simulink model "RequirementsTable"  (R2022b)
settings: Solver=FixedStepAuto  StartTime=0.0  StopTime=10.0  FixedStep=1e-3  RelTol=1e-3  EnableMultiTasking=on
settings Model: DVExtractedSubsystem=Requirements Table  Creator=coler  LastModifiedBy=coler
settings SolverCC: AlgebraicLoopSolver=TrustRegion
settings OptimizationCC: EnhancedBackFolding=on  PassReuseOutputArgsAs=Individual arguments  ZeroExternalMemoryAtStartup=off  ZeroInternalMemoryAtStartup=off  MaxStackSize=64  OptimizeBlockOrder=speed  DifferentSizesBufferReuse=on  OptimizationCustomize=off  EfficientTunableParamExpr=on
settings DebuggingCC: ParameterTunabilityLossMsg=error  UnconnectedInputMsg=warning  UnconnectedOutputMsg=warning  UnconnectedLineMsg=warning  FrameProcessingCompatibilityMsg=none  SFMachineParentedDataDiag=warning
settings HardwareCC: ProdBitPerPointer=32  ProdBitPerSizeT=32  ProdBitPerPtrDiffT=32  ProdLargestAtomicInteger=Long  ProdLargestAtomicFloat=Double  ProdWordSize=32  ProdHWDeviceType=ARM Compatible->ARM Cortex
settings ModelReferenceCC: EnableRefExpFcnMdlSchedulingChecks=on
settings SFSimCC: MATLABDynamicMemAlloc=off
settings RTWCC: Description=Embedded Coder  SystemTargetFile=ert.tlc  HardwareBoard=NXP FRDM-K64F  TemplateMakefile=ert_default_tmf  Toolchain=GNU Tools for ARM Embedded Processors
settings CodeAppCC: ForceParamTrailComments=on  IgnoreCustomStorageClasses=off  OperatorAnnotations=on  SimulinkDataObjDesc=on  SFDataObjDesc=on  InsertBlockDesc=on
settings ERTTargetCC: ExtMode=on  ExtModeTransport=4  ExtModeMexFile=sendToCommService  ExtModeMexArgs='RA_Modes' 0

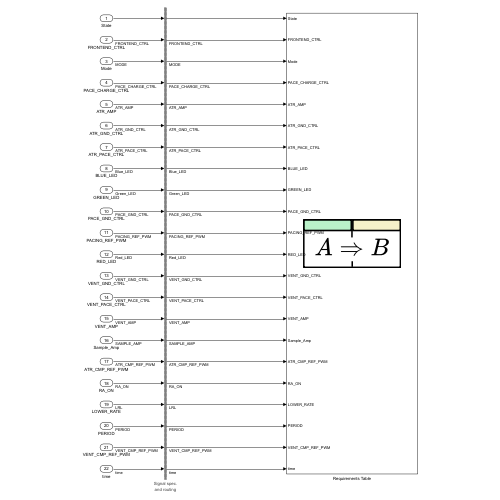
[thumbnail: Simulink's stored preview of the top-level diagram]
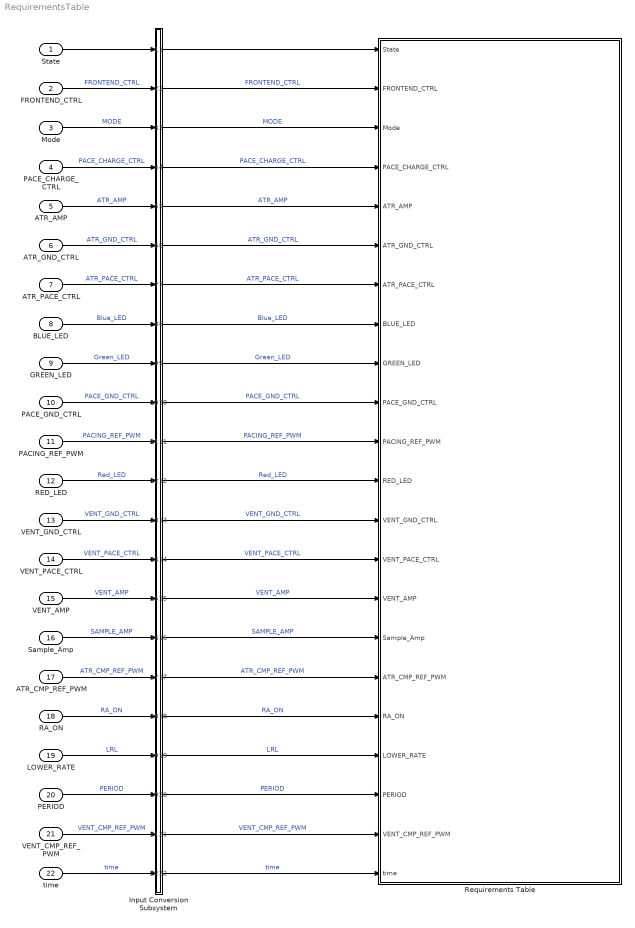
== system RequirementsTable ==
  State : Inport  OutDataTypeStr=double  PortDimensions=[1]  SampleTime=[-1, 0]  Interpolate=off
  FRONTEND_CTRL : Inport  Port=2  OutDataTypeStr=double  PortDimensions=[1]  SampleTime=0.001  Interpolate=off
  Mode : Inport  Port=3  OutDataTypeStr=double  PortDimensions=[1]  SampleTime=[-1, 0]  Interpolate=off
  PACE_CHARGE_CTRL : Inport  Port=4  OutDataTypeStr=double  PortDimensions=[1]  SampleTime=0.001  Interpolate=off
  ATR_AMP : Inport  Port=5  OutDataTypeStr=double  PortDimensions=[1]  SampleTime=[-1, 0]  Interpolate=off
  ATR_GND_CTRL : Inport  Port=6  OutDataTypeStr=double  PortDimensions=[1]  SampleTime=0.001  Interpolate=off
  ATR_PACE_CTRL : Inport  Port=7  OutDataTypeStr=double  PortDimensions=[1]  SampleTime=0.001  Interpolate=off
  BLUE_LED : Inport  Port=8  OutDataTypeStr=boolean  PortDimensions=[1]  SampleTime=0.001  Interpolate=off
  GREEN_LED : Inport  Port=9  OutDataTypeStr=boolean  PortDimensions=[1]  SampleTime=0.001  Interpolate=off
  PACE_GND_CTRL : Inport  Port=10  OutDataTypeStr=double  PortDimensions=[1]  SampleTime=0.001  Interpolate=off
  PACING_REF_PWM : Inport  Port=11  OutDataTypeStr=double  PortDimensions=[1]  SampleTime=0.001  Interpolate=off
  RED_LED : Inport  Port=12  OutDataTypeStr=boolean  PortDimensions=[1]  SampleTime=0.001  Interpolate=off
  VENT_GND_CTRL : Inport  Port=13  OutDataTypeStr=double  PortDimensions=[1]  SampleTime=0.001  Interpolate=off
  VENT_PACE_CTRL : Inport  Port=14  OutDataTypeStr=double  PortDimensions=[1]  SampleTime=0.001  Interpolate=off
  VENT_AMP : Inport  Port=15  OutDataTypeStr=double  PortDimensions=[1]  SampleTime=[-1, 0]  Interpolate=off
  Sample_Amp : Inport  Port=16  OutDataTypeStr=double  PortDimensions=[1]  SampleTime=[-1, 0]  Interpolate=off
  ATR_CMP_REF_PWM : Inport  Port=17  OutDataTypeStr=double  PortDimensions=[1]  SampleTime=0.001  Interpolate=off
  RA_ON : Inport  Port=18  OutDataTypeStr=boolean  PortDimensions=[1]  SampleTime=[-1, 0]  Interpolate=off
  LOWER_RATE : Inport  Port=19  OutDataTypeStr=double  PortDimensions=[1]  SampleTime=[-1, 0]  Interpolate=off
  PERIOD : Inport  Port=20  OutDataTypeStr=double  PortDimensions=[1]  SampleTime=0.001  Interpolate=off
  VENT_CMP_REF_PWM : Inport  Port=21  OutDataTypeStr=double  PortDimensions=[1]  SampleTime=0.001  Interpolate=off
  time : Inport  Port=22  OutDataTypeStr=double  PortDimensions=[1]  Interpolate=off
  Input Conversion Subsystem : Subsystem  Tag=__SLT_ICS__  Description=|
      | Signal spec.
      | and routing
      settings: AttributesFormatString=%<Description>
  Requirements Table : Requirements Table  TreatAsAtomicUnit=on
  wires:
  State/1 -> Input Conversion Subsystem/1(Inport_1)
  FRONTEND_CTRL/1 -> Input Conversion Subsystem/2(Inport_2)  "FRONTEND_CTRL"
  Mode/1 -> Input Conversion Subsystem/3(Inport_3)  "MODE"
  PACE_CHARGE_CTRL/1 -> Input Conversion Subsystem/4(Inport_4)  "PACE_CHARGE_CTRL"
  ATR_AMP/1 -> Input Conversion Subsystem/5(Inport_5)  "ATR_AMP"
  ATR_GND_CTRL/1 -> Input Conversion Subsystem/6(Inport_6)  "ATR_GND_CTRL"
  ATR_PACE_CTRL/1 -> Input Conversion Subsystem/7(Inport_7)  "ATR_PACE_CTRL"
  BLUE_LED/1 -> Input Conversion Subsystem/8(Inport_8)  "Blue_LED"
  GREEN_LED/1 -> Input Conversion Subsystem/9(Inport_9)  "Green_LED"
  PACE_GND_CTRL/1 -> Input Conversion Subsystem/10(Inport_10)  "PACE_GND_CTRL"
  PACING_REF_PWM/1 -> Input Conversion Subsystem/11(Inport_11)  "PACING_REF_PWM"
  RED_LED/1 -> Input Conversion Subsystem/12(Inport_12)  "Red_LED"
  VENT_GND_CTRL/1 -> Input Conversion Subsystem/13(Inport_13)  "VENT_GND_CTRL"
  VENT_PACE_CTRL/1 -> Input Conversion Subsystem/14(Inport_14)  "VENT_PACE_CTRL"
  VENT_AMP/1 -> Input Conversion Subsystem/15(Inport_15)  "VENT_AMP"
  Sample_Amp/1 -> Input Conversion Subsystem/16(Inport_16)  "SAMPLE_AMP"
  ATR_CMP_REF_PWM/1 -> Input Conversion Subsystem/17(Inport_17)  "ATR_CMP_REF_PWM"
  RA_ON/1 -> Input Conversion Subsystem/18(Inport_18)  "RA_ON"
  LOWER_RATE/1 -> Input Conversion Subsystem/19(Inport_19)  "LRL"
  PERIOD/1 -> Input Conversion Subsystem/20(Inport_20)  "PERIOD"
  VENT_CMP_REF_PWM/1 -> Input Conversion Subsystem/21(Inport_21)  "VENT_CMP_REF_PWM"
  time/1 -> Input Conversion Subsystem/22(Inport_22)  "time"
  Input Conversion Subsystem/1(Outport_1) -> Requirements Table/1(State)
  Input Conversion Subsystem/2(Outport_2) -> Requirements Table/2(FRONTEND_CTRL)  "FRONTEND_CTRL"
  Input Conversion Subsystem/3(Outport_3) -> Requirements Table/3(Mode)  "MODE"
  Input Conversion Subsystem/4(Outport_4) -> Requirements Table/4(PACE_CHARGE_CTRL)  "PACE_CHARGE_CTRL"
  Input Conversion Subsystem/5(Outport_5) -> Requirements Table/5(ATR_AMP)  "ATR_AMP"
  Input Conversion Subsystem/6(Outport_6) -> Requirements Table/6(ATR_GND_CTRL)  "ATR_GND_CTRL"
  Input Conversion Subsystem/7(Outport_7) -> Requirements Table/7(ATR_PACE_CTRL)  "ATR_PACE_CTRL"
  Input Conversion Subsystem/8(Outport_8) -> Requirements Table/8(BLUE_LED)  "Blue_LED"
  Input Conversion Subsystem/9(Outport_9) -> Requirements Table/9(GREEN_LED)  "Green_LED"
  Input Conversion Subsystem/10(Outport_10) -> Requirements Table/10(PACE_GND_CTRL)  "PACE_GND_CTRL"
  Input Conversion Subsystem/11(Outport_11) -> Requirements Table/11(PACING_REF_PWM)  "PACING_REF_PWM"
  Input Conversion Subsystem/12(Outport_12) -> Requirements Table/12(RED_LED)  "Red_LED"
  Input Conversion Subsystem/13(Outport_13) -> Requirements Table/13(VENT_GND_CTRL)  "VENT_GND_CTRL"
  Input Conversion Subsystem/14(Outport_14) -> Requirements Table/14(VENT_PACE_CTRL)  "VENT_PACE_CTRL"
  Input Conversion Subsystem/15(Outport_15) -> Requirements Table/15(VENT_AMP)  "VENT_AMP"
  Input Conversion Subsystem/16(Outport_16) -> Requirements Table/16(Sample_Amp)  "SAMPLE_AMP"
  Input Conversion Subsystem/17(Outport_17) -> Requirements Table/17(ATR_CMP_REF_PWM)  "ATR_CMP_REF_PWM"
  Input Conversion Subsystem/18(Outport_18) -> Requirements Table/18(RA_ON)  "RA_ON"
  Input Conversion Subsystem/19(Outport_19) -> Requirements Table/19(LOWER_RATE)  "LRL"
  Input Conversion Subsystem/20(Outport_20) -> Requirements Table/20(PERIOD)  "PERIOD"
  Input Conversion Subsystem/21(Outport_21) -> Requirements Table/21(VENT_CMP_REF_PWM)  "VENT_CMP_REF_PWM"
  Input Conversion Subsystem/22(Outport_22) -> Requirements Table/22(time)  "time"

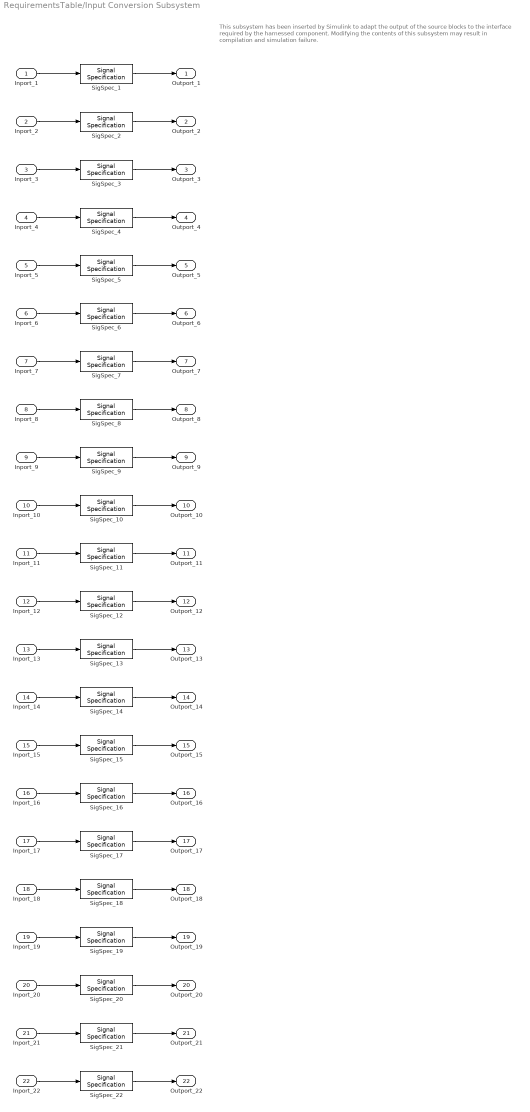
== system RequirementsTable/Input Conversion Subsystem ==
  note: This subsystem has been inserted by Simulink to adapt the output of the source blocks to the interface required by the harnessed component.
      |  Modifying the contents of this subsystem may result in compilation and simulation failure.
  Inport_1 : Inport
  Inport_2 : Inport  Port=2
  Inport_3 : Inport  Port=3
  Inport_4 : Inport  Port=4
  Inport_5 : Inport  Port=5
  Inport_6 : Inport  Port=6
  Inport_7 : Inport  Port=7
  Inport_8 : Inport  Port=8
  Inport_9 : Inport  Port=9
  Inport_10 : Inport  Port=10
  Inport_11 : Inport  Port=11
  Inport_12 : Inport  Port=12
  Inport_13 : Inport  Port=13
  Inport_14 : Inport  Port=14
  Inport_15 : Inport  Port=15
  Inport_16 : Inport  Port=16
  Inport_17 : Inport  Port=17
  Inport_18 : Inport  Port=18
  Inport_19 : Inport  Port=19
  Inport_20 : Inport  Port=20
  Inport_21 : Inport  Port=21
  Inport_22 : Inport  Port=22
  SigSpec_{1,3,5,15..16,19} (6 alike) : SignalSpecification  OutDataTypeStr=double  Dimensions=[1]  SampleTime=[-1, 0]
  SigSpec_{2,4,6..7,10..11,13..14,17,20..21} (11 alike) : SignalSpecification  OutDataTypeStr=double  Dimensions=[1]  SampleTime=0.001
  SigSpec_12 : SignalSpecification  OutDataTypeStr=boolean  Dimensions=[1]  SampleTime=0.001
  SigSpec_18 : SignalSpecification  OutDataTypeStr=boolean  Dimensions=[1]  SampleTime=[-1, 0]
  SigSpec_22 : SignalSpecification  OutDataTypeStr=double  Dimensions=[1]
  SigSpec_8 : SignalSpecification  OutDataTypeStr=boolean  Dimensions=[1]  SampleTime=0.001
  SigSpec_9 : SignalSpecification  OutDataTypeStr=boolean  Dimensions=[1]  SampleTime=0.001
  Outport_1 : Outport
  Outport_2 : Outport  Port=2
  Outport_3 : Outport  Port=3
  Outport_4 : Outport  Port=4
  Outport_5 : Outport  Port=5
  Outport_6 : Outport  Port=6
  Outport_7 : Outport  Port=7
  Outport_8 : Outport  Port=8
  Outport_9 : Outport  Port=9
  Outport_10 : Outport  Port=10
  Outport_11 : Outport  Port=11
  Outport_12 : Outport  Port=12
  Outport_13 : Outport  Port=13
  Outport_14 : Outport  Port=14
  Outport_15 : Outport  Port=15
  Outport_16 : Outport  Port=16
  Outport_17 : Outport  Port=17
  Outport_18 : Outport  Port=18
  Outport_19 : Outport  Port=19
  Outport_20 : Outport  Port=20
  Outport_21 : Outport  Port=21
  Outport_22 : Outport  Port=22
  wires:
  SigSpec_1/1 -> Outport_1/1
  Inport_1/1 -> SigSpec_1/1
  SigSpec_2/1 -> Outport_2/1
  Inport_2/1 -> SigSpec_2/1
  SigSpec_3/1 -> Outport_3/1
  Inport_3/1 -> SigSpec_3/1
  SigSpec_4/1 -> Outport_4/1
  Inport_4/1 -> SigSpec_4/1
  SigSpec_5/1 -> Outport_5/1
  Inport_5/1 -> SigSpec_5/1
  SigSpec_6/1 -> Outport_6/1
  Inport_6/1 -> SigSpec_6/1
  SigSpec_7/1 -> Outport_7/1
  Inport_7/1 -> SigSpec_7/1
  SigSpec_8/1 -> Outport_8/1
  Inport_8/1 -> SigSpec_8/1
  SigSpec_9/1 -> Outport_9/1
  Inport_9/1 -> SigSpec_9/1
  SigSpec_10/1 -> Outport_10/1
  Inport_10/1 -> SigSpec_10/1
  SigSpec_11/1 -> Outport_11/1
  Inport_11/1 -> SigSpec_11/1
  SigSpec_12/1 -> Outport_12/1
  Inport_12/1 -> SigSpec_12/1
  SigSpec_13/1 -> Outport_13/1
  Inport_13/1 -> SigSpec_13/1
  SigSpec_14/1 -> Outport_14/1
  Inport_14/1 -> SigSpec_14/1
  SigSpec_15/1 -> Outport_15/1
  Inport_15/1 -> SigSpec_15/1
  SigSpec_16/1 -> Outport_16/1
  Inport_16/1 -> SigSpec_16/1
  SigSpec_17/1 -> Outport_17/1
  Inport_17/1 -> SigSpec_17/1
  SigSpec_18/1 -> Outport_18/1
  Inport_18/1 -> SigSpec_18/1
  SigSpec_19/1 -> Outport_19/1
  Inport_19/1 -> SigSpec_19/1
  SigSpec_20/1 -> Outport_20/1
  Inport_20/1 -> SigSpec_20/1
  SigSpec_21/1 -> Outport_21/1
  Inport_21/1 -> SigSpec_21/1
  SigSpec_22/1 -> Outport_22/1
  Inport_22/1 -> SigSpec_22/1

== stateflow chart RequirementsTable/Requirements Table ==
  (default) -> (junction 1073748085)
  (junction 1073748085) -> (junction 1073748086) : {
      | % SF_REQ_REV_07
      | }
  (junction 1073748086) -> (junction 1073748088) : {
      | % HEADER_ASSIGNMENTS
      |
      | }
  (junction 1073748088) -> (junction 1073748090) : {
      | % START_A_28
      | }
  (junction 1073748090) -> (junction 1073748092) : {
      | }
  (junction 1073748092) -> (junction 1073748094)
  (junction 1073748094) -> (junction 1073748096) : {
      | }
  (junction 1073748096) -> (junction 1073748098) : {
      | % END_A_28
      | }
  (junction 1073748098) -> (junction 1073748100) : {
      | % START_R_1
      | }
  (junction 1073748100) -> (junction 1073748102) : {
      | }
  (junction 1073748102) -> (junction 1073748104)
  (junction 1073748104) -> (junction 1073748106) [order 1] : [(((RA_ON) == (0))) && (((Mode) == (1))) && (((State) == (0)))]
  (junction 1073748104) -> (junction 1073748112) [order 2]
  (junction 1073748106) -> (junction 1073748108) : {
      | reqtable_postcondition((((PACE_CHARGE_CTRL) == (1))) && (ATR_PACE_CTRL == 0) && (((PACING_REF_PWM ) == (ATR_AMP))) && (((PACE_CHARGE_CTRL) == (1))) && (((PACE_GND_CTRL) == (1))) && (ATR_GND_CTRL == 1) && (((RED_LED) == (0))) && (((GREEN_LED) == (0))) && (((BLUE_LED) == (0))) && (time-oldTime / (60*1000) >= LOWER_RATE), 'R:1');
      |
      | }
  (junction 1073748108) -> (junction 1073748110) : {
      | }
  (junction 1073748110) -> (junction 1073748112)
  (junction 1073748112) -> (junction 1073748114)
  (junction 1073748114) -> (junction 1073748116) : {
      | % END_R_1
      | }
  (junction 1073748116) -> (junction 1073748118) : {
      | % START_R_82
      | }
  (junction 1073748118) -> (junction 1073748120) : {
      | }
  (junction 1073748120) -> (junction 1073748122)
  (junction 1073748122) -> (junction 1073748124) [order 1] : [(((RA_ON) == (1))) && (((Mode) == (1))) && (((State) == (0)))]
  (junction 1073748122) -> (junction 1073748130) [order 2]
  (junction 1073748124) -> (junction 1073748126) : {
      | reqtable_postcondition((((PACE_CHARGE_CTRL) == (1))) && (ATR_PACE_CTRL == 0) && (((PACING_REF_PWM ) == (ATR_AMP))) && (((PACE_CHARGE_CTRL) == (1))) && (((PACE_GND_CTRL) == (1))) && (ATR_GND_CTRL == 1) && (((RED_LED) == (0))) && (((GREEN_LED) == (0))) && (((BLUE_LED) == (0))) && (time-oldTime >= PERIOD-5), 'R:2');
      |
      | }
  (junction 1073748126) -> (junction 1073748128) : {
      | }
  (junction 1073748128) -> (junction 1073748130)
  (junction 1073748130) -> (junction 1073748132)
  (junction 1073748132) -> (junction 1073748134) : {
      | % END_R_82
      | }
  (junction 1073748134) -> (junction 1073748136) : {
      | % START_R_7
      | }
  (junction 1073748136) -> (junction 1073748138) : {
      | }
  (junction 1073748138) -> (junction 1073748140)
  (junction 1073748140) -> (junction 1073748142) [order 1] : [(((RA_ON) == (0))) && (((Mode) == (1))) && (((State) == (1)))]
  (junction 1073748140) -> (junction 1073748148) [order 2]
  (junction 1073748142) -> (junction 1073748144) : {
      | reqtable_postcondition((((PACE_CHARGE_CTRL) == (0))) && (ATR_PACE_CTRL == 1) && (((PACING_REF_PWM ) == (ATR_AMP))) && (((PACE_CHARGE_CTRL) == (0))) && (((PACE_GND_CTRL) == (1))) && (ATR_GND_CTRL == 0) && (((RED_LED) == (1))) && (((GREEN_LED) == (0))) && (((BLUE_LED) == (0))) && (time-oldTime / (60*1000) >= LOWER_RATE), 'R:3');
      |
      | }
  (junction 1073748144) -> (junction 1073748146) : {
      | }
  (junction 1073748146) -> (junction 1073748148)
  (junction 1073748148) -> (junction 1073748150)
  (junction 1073748150) -> (junction 1073748152) : {
      | % END_R_7
      | }
  (junction 1073748152) -> (junction 1073748154) : {
      | % START_R_88
      | }
  (junction 1073748154) -> (junction 1073748156) : {
      | }
  (junction 1073748156) -> (junction 1073748158)
  (junction 1073748158) -> (junction 1073748160) [order 1] : [(((RA_ON) == (1))) && (((Mode) == (1))) && (((State) == (1)))]
  (junction 1073748158) -> (junction 1073748166) [order 2]
  (junction 1073748160) -> (junction 1073748162) : {
      | reqtable_postcondition((((PACE_CHARGE_CTRL) == (0))) && (ATR_PACE_CTRL == 1) && (((PACING_REF_PWM ) == (ATR_AMP))) && (((PACE_CHARGE_CTRL) == (0))) && (((PACE_GND_CTRL) == (1))) && (ATR_GND_CTRL == 0) && (((RED_LED) == (1))) && (((GREEN_LED) == (0))) && (((BLUE_LED) == (0))) && (time-oldTime >= PERIOD-5), 'R:4');
      |
      | }
  (junction 1073748162) -> (junction 1073748164) : {
      | }
  (junction 1073748164) -> (junction 1073748166)
  (junction 1073748166) -> (junction 1073748168)
  (junction 1073748168) -> (junction 1073748170) : {
      | % END_R_88
      | }
  (junction 1073748170) -> (junction 1073748172) : {
      | % START_R_10
      | }
  (junction 1073748172) -> (junction 1073748174) : {
      | }
  (junction 1073748174) -> (junction 1073748176)
  (junction 1073748176) -> (junction 1073748178) [order 1] : [(((RA_ON) == (0))) && (((Mode) == (3))) && (((State) == (0)))]
  (junction 1073748176) -> (junction 1073748184) [order 2]
  (junction 1073748178) -> (junction 1073748180) : {
      | reqtable_postcondition((((PACE_CHARGE_CTRL) == (1))) && (VENT_PACE_CTRL == 0) && (((PACING_REF_PWM ) == (VENT_AMP))) && (((PACE_CHARGE_CTRL) == (1))) && (((PACE_GND_CTRL) == (1))) && (VENT_GND_CTRL == 1) && (((RED_LED) == (0))) && (((GREEN_LED) == (0))) && (((BLUE_LED) == (0))) && (time-oldTime / (60*1000) >= LOWER_RATE), 'R:5');
      |
      | }
  (junction 1073748180) -> (junction 1073748182) : {
      | }
  (junction 1073748182) -> (junction 1073748184)
  (junction 1073748184) -> (junction 1073748186)
  (junction 1073748186) -> (junction 1073748188) : {
      | % END_R_10
      | }
  (junction 1073748188) -> (junction 1073748190) : {
      | % START_R_85
      | }
  (junction 1073748190) -> (junction 1073748192) : {
      | }
  (junction 1073748192) -> (junction 1073748194)
  (junction 1073748194) -> (junction 1073748196) [order 1] : [(((RA_ON) == (1))) && (((Mode) == (3))) && (((State) == (0)))]
  (junction 1073748194) -> (junction 1073748202) [order 2]
  (junction 1073748196) -> (junction 1073748198) : {
      | reqtable_postcondition((((PACE_CHARGE_CTRL) == (1))) && (VENT_PACE_CTRL == 0) && (((PACING_REF_PWM ) == (VENT_AMP))) && (((PACE_CHARGE_CTRL) == (1))) && (((PACE_GND_CTRL) == (1))) && (VENT_GND_CTRL == 1) && (((RED_LED) == (0))) && (((GREEN_LED) == (0))) && (((BLUE_LED) == (0))) && (time-oldTime >= PERIOD-5), 'R:6');
      |
      | }
  (junction 1073748198) -> (junction 1073748200) : {
      | }
  (junction 1073748200) -> (junction 1073748202)
  (junction 1073748202) -> (junction 1073748204)
  (junction 1073748204) -> (junction 1073748206) : {
      | % END_R_85
      | }
  (junction 1073748206) -> (junction 1073748208) : {
      | % START_R_13
      | }
  (junction 1073748208) -> (junction 1073748210) : {
      | }
  (junction 1073748210) -> (junction 1073748212)
  (junction 1073748212) -> (junction 1073748214) [order 1] : [(((RA_ON) == (0))) && (((Mode) == (3))) && (((State) == (1)))]
  (junction 1073748212) -> (junction 1073748220) [order 2]
  (junction 1073748214) -> (junction 1073748216) : {
      | reqtable_postcondition((((PACE_CHARGE_CTRL) == (0))) && (VENT_PACE_CTRL == 1) && (((PACING_REF_PWM ) == (VENT_AMP))) && (((PACE_CHARGE_CTRL) == (0))) && (((PACE_GND_CTRL) == (1))) && (VENT_GND_CTRL == 0) && (((RED_LED) == (0))) && (((GREEN_LED) == (1))) && (((BLUE_LED) == (0))) && (time-oldTime / (60*1000) >= LOWER_RATE), 'R:7');
      |
      | }
  (junction 1073748216) -> (junction 1073748218) : {
      | }
  (junction 1073748218) -> (junction 1073748220)
  (junction 1073748220) -> (junction 1073748222)
  (junction 1073748222) -> (junction 1073748224) : {
      | % END_R_13
      | }
  (junction 1073748224) -> (junction 1073748226) : {
      | % START_R_91
      | }
  (junction 1073748226) -> (junction 1073748228) : {
      | }
  (junction 1073748228) -> (junction 1073748230)
  (junction 1073748230) -> (junction 1073748232) [order 1] : [(((RA_ON) == (1))) && (((Mode) == (3))) && (((State) == (1)))]
  (junction 1073748230) -> (junction 1073748238) [order 2]
  (junction 1073748232) -> (junction 1073748234) : {
      | reqtable_postcondition((((PACE_CHARGE_CTRL) == (0))) && (VENT_PACE_CTRL == 1) && (((PACING_REF_PWM ) == (VENT_AMP))) && (((PACE_CHARGE_CTRL) == (0))) && (((PACE_GND_CTRL) == (1))) && (VENT_GND_CTRL == 0) && (((RED_LED) == (0))) && (((GREEN_LED) == (1))) && (((BLUE_LED) == (0))) && (time-oldTime >= PERIOD-5), 'R:8');
      |
      | }
  (junction 1073748234) -> (junction 1073748236) : {
      | }
  (junction 1073748236) -> (junction 1073748238)
  (junction 1073748238) -> (junction 1073748240)
  (junction 1073748240) -> (junction 1073748242) : {
      | % END_R_91
      | }
  (junction 1073748242) -> (junction 1073748244) : {
      | % START_R_16
      | }
  (junction 1073748244) -> (junction 1073748246) : {
      | }
  (junction 1073748246) -> (junction 1073748248)
  (junction 1073748248) -> (junction 1073748250) [order 1] : [(((RA_ON) == (0))) && (((Mode) == (2))) && (((State) == (0))) && (FRONTEND_CTRL == 1)]
  (junction 1073748248) -> (junction 1073748256) [order 2]
  (junction 1073748250) -> (junction 1073748252) : {
      | reqtable_postcondition((((PACE_CHARGE_CTRL) == (1))) && (ATR_PACE_CTRL == 0) && (((PACING_REF_PWM ) == (ATR_AMP))) && (((PACE_CHARGE_CTRL) == (1))) && (((PACE_GND_CTRL) == (1))) && (ATR_GND_CTRL == 1) && (((RED_LED) == (0))) && (((GREEN_LED) == (0))) && (((BLUE_LED) == (0))) && (ATR_CMP_REF_PWM == Sample_Amp) && (time-oldTime / (60*1000) >= LOWER_RATE), 'R:9');
      |
      | }
  (junction 1073748252) -> (junction 1073748254) : {
      | }
  (junction 1073748254) -> (junction 1073748256)
  (junction 1073748256) -> (junction 1073748258)
  (junction 1073748258) -> (junction 1073748260) : {
      | % END_R_16
      | }
  (junction 1073748260) -> (junction 1073748262) : {
      | % START_R_94
      | }
  (junction 1073748262) -> (junction 1073748264) : {
      | }
  (junction 1073748264) -> (junction 1073748266)
  (junction 1073748266) -> (junction 1073748268) [order 1] : [(((RA_ON) == (1))) && (((Mode) == (2))) && (((State) == (0))) && (FRONTEND_CTRL == 1)]
  (junction 1073748266) -> (junction 1073748274) [order 2]
  (junction 1073748268) -> (junction 1073748270) : {
      | reqtable_postcondition((((PACE_CHARGE_CTRL) == (1))) && (ATR_PACE_CTRL == 0) && (((PACING_REF_PWM ) == (ATR_AMP))) && (((PACE_CHARGE_CTRL) == (1))) && (((PACE_GND_CTRL) == (1))) && (ATR_GND_CTRL == 1) && (((RED_LED) == (0))) && (((GREEN_LED) == (0))) && (((BLUE_LED) == (0))) && (ATR_CMP_REF_PWM == Sample_Amp) && (time-oldTime >= PERIOD-5), 'R:10');
      |
      | }
  (junction 1073748270) -> (junction 1073748272) : {
      | }
  (junction 1073748272) -> (junction 1073748274)
  (junction 1073748274) -> (junction 1073748276)
  (junction 1073748276) -> (junction 1073748278) : {
      | % END_R_94
      | }
  (junction 1073748278) -> (junction 1073748280) : {
      | % START_R_19
      | }
  (junction 1073748280) -> (junction 1073748282) : {
      | }
  (junction 1073748282) -> (junction 1073748284)
  (junction 1073748284) -> (junction 1073748286) [order 1] : [(((RA_ON) == (0))) && (((Mode) == (2))) && (((State) == (1)))]
  (junction 1073748284) -> (junction 1073748292) [order 2]
  (junction 1073748286) -> (junction 1073748288) : {
      | reqtable_postcondition((((PACE_CHARGE_CTRL) == (0))) && (ATR_PACE_CTRL == 1) && (((PACING_REF_PWM ) == (ATR_AMP))) && (((PACE_CHARGE_CTRL) == (0))) && (((PACE_GND_CTRL) == (1))) && (ATR_GND_CTRL == 0) && (((RED_LED) == (0))) && (((GREEN_LED) == (0))) && (((BLUE_LED) == (0))) && (ATR_CMP_REF_PWM == Sample_Amp) && (time-oldTime / (60*1000) >= LOWER_RATE), 'R:11');
      |
      | }
  (junction 1073748288) -> (junction 1073748290) : {
      | }
  (junction 1073748290) -> (junction 1073748292)
  (junction 1073748292) -> (junction 1073748294)
  (junction 1073748294) -> (junction 1073748296) : {
      | % END_R_19
      | }
  (junction 1073748296) -> (junction 1073748298) : {
      | % START_R_97
      | }
  (junction 1073748298) -> (junction 1073748300) : {
      | }
  (junction 1073748300) -> (junction 1073748302)
  (junction 1073748302) -> (junction 1073748304) [order 1] : [(((RA_ON) == (1))) && (((Mode) == (2))) && (((State) == (1)))]
  (junction 1073748302) -> (junction 1073748310) [order 2]
  (junction 1073748304) -> (junction 1073748306) : {
      | reqtable_postcondition((((PACE_CHARGE_CTRL) == (0))) && (ATR_PACE_CTRL == 1) && (((PACING_REF_PWM ) == (ATR_AMP))) && (((PACE_CHARGE_CTRL) == (0))) && (((PACE_GND_CTRL) == (1))) && (ATR_GND_CTRL == 0) && (((RED_LED) == (0))) && (((GREEN_LED) == (0))) && (((BLUE_LED) == (0))) && (ATR_CMP_REF_PWM == Sample_Amp) && (time-oldTime >= PERIOD-5), 'R:12');
      |
      | }
  (junction 1073748306) -> (junction 1073748308) : {
      | }
  (junction 1073748308) -> (junction 1073748310)
  (junction 1073748310) -> (junction 1073748312)
  (junction 1073748312) -> (junction 1073748314) : {
      | % END_R_97
      | }
  (junction 1073748314) -> (junction 1073748316) : {
      | % START_R_22
      | }
  (junction 1073748316) -> (junction 1073748318) : {
      | }
  (junction 1073748318) -> (junction 1073748320)
  (junction 1073748320) -> (junction 1073748322) [order 1] : [(((RA_ON) == (0))) && (((Mode) == (4))) && (((State) == (0))) && (FRONTEND_CTRL == 1)]
  (junction 1073748320) -> (junction 1073748328) [order 2]
  (junction 1073748322) -> (junction 1073748324) : {
      | reqtable_postcondition((((PACE_CHARGE_CTRL) == (1))) && (VENT_PACE_CTRL == 0) && (((PACING_REF_PWM ) == (VENT_AMP))) && (((PACE_CHARGE_CTRL) == (1))) && (((PACE_GND_CTRL) == (1))) && (VENT_GND_CTRL == 1) && (((RED_LED) == (0))) && (((GREEN_LED) == (0))) && (((BLUE_LED) == (0))) && (VENT_CMP_REF_PWM == Sample_Amp) && (time-oldTime / (60*1000) >= LOWER_RATE), 'R:13');
      |
      | }
  (junction 1073748324) -> (junction 1073748326) : {
      | }
  (junction 1073748326) -> (junction 1073748328)
  (junction 1073748328) -> (junction 1073748330)
  (junction 1073748330) -> (junction 1073748332) : {
      | % END_R_22
      | }
  (junction 1073748332) -> (junction 1073748334) : {
      | % START_R_100
      | }
  (junction 1073748334) -> (junction 1073748336) : {
      | }
  (junction 1073748336) -> (junction 1073748338)
  (junction 1073748338) -> (junction 1073748340) [order 1] : [(((RA_ON) == (1))) && (((Mode) == (4))) && (((State) == (0))) && (FRONTEND_CTRL == 1)]
  (junction 1073748338) -> (junction 1073748346) [order 2]
  (junction 1073748340) -> (junction 1073748342) : {
      | reqtable_postcondition((((PACE_CHARGE_CTRL) == (1))) && (VENT_PACE_CTRL == 0) && (((PACING_REF_PWM ) == (VENT_AMP))) && (((PACE_CHARGE_CTRL) == (1))) && (((PACE_GND_CTRL) == (1))) && (VENT_GND_CTRL == 1) && (((RED_LED) == (0))) && (((GREEN_LED) == (0))) && (((BLUE_LED) == (0))) && (VENT_CMP_REF_PWM == Sample_Amp) && (time-oldTime >= PERIOD-5), 'R:14');
      |
      | }
  (junction 1073748342) -> (junction 1073748344) : {
      | }
  (junction 1073748344) -> (junction 1073748346)
  (junction 1073748346) -> (junction 1073748348)
  (junction 1073748348) -> (junction 1073748350) : {
      | % END_R_100
      | }
  (junction 1073748350) -> (junction 1073748352) : {
      | % START_R_25
      | }
  (junction 1073748352) -> (junction 1073748354) : {
      | }
  (junction 1073748354) -> (junction 1073748356)
  (junction 1073748356) -> (junction 1073748358) [order 1] : [(((RA_ON) == (0))) && (((Mode) == (4))) && (((State) == (1)))]
  (junction 1073748356) -> (junction 1073748364) [order 2]
  (junction 1073748358) -> (junction 1073748360) : {
      | reqtable_postcondition((((PACE_CHARGE_CTRL) == (0))) && (VENT_PACE_CTRL == 1) && (((PACING_REF_PWM ) == (VENT_AMP))) && (((PACE_CHARGE_CTRL) == (0))) && (((PACE_GND_CTRL) == (1))) && (VENT_GND_CTRL == 0) && (((RED_LED) == (0))) && (((GREEN_LED) == (1))) && (((BLUE_LED) == (0))) && (VENT_CMP_REF_PWM == Sample_Amp) && (time-oldTime / (60*1000) >= LOWER_RATE), 'R:15');
      |
      | }
  (junction 1073748360) -> (junction 1073748362) : {
      | }
  (junction 1073748362) -> (junction 1073748364)
  (junction 1073748364) -> (junction 1073748366)
  (junction 1073748366) -> (junction 1073748368) : {
      | % END_R_25
      | }
  (junction 1073748368) -> (junction 1073748370) : {
      | % START_R_103
      | }
  (junction 1073748370) -> (junction 1073748372) : {
      | }
  (junction 1073748372) -> (junction 1073748374)
  (junction 1073748374) -> (junction 1073748376) [order 1] : [(((RA_ON) == (1))) && (((Mode) == (4))) && (((State) == (1)))]
  (junction 1073748374) -> (junction 1073748382) [order 2]
  (junction 1073748376) -> (junction 1073748378) : {
      | reqtable_postcondition((((PACE_CHARGE_CTRL) == (0))) && (VENT_PACE_CTRL == 1) && (((PACING_REF_PWM ) == (VENT_AMP))) && (((PACE_CHARGE_CTRL) == (0))) && (((PACE_GND_CTRL) == (1))) && (VENT_GND_CTRL == 0) && (((RED_LED) == (0))) && (((GREEN_LED) == (1))) && (((BLUE_LED) == (0))) && (VENT_CMP_REF_PWM == Sample_Amp) && (time-oldTime >= PERIOD-5), 'R:16');
      |
      | }
  (junction 1073748378) -> (junction 1073748380) : {
      | }
  (junction 1073748380) -> (junction 1073748382)
  (junction 1073748382) -> (junction 1073748384)
  (junction 1073748384) -> (junction 1073748386) : {
      | % END_R_103
      | }
  data: State input; FRONTEND_CTRL input; Mode input; PACE_CHARGE_CTRL input; ATR_AMP input; ATR_GND_CTRL input; ATR_PACE_CTRL input; BLUE_LED input; GREEN_LED input; PACE_GND_CTRL input; PACING_REF_PWM input; RED_LED input; VENT_GND_CTRL input; VENT_PACE_CTRL input; VENT_AMP input; Sample_Amp input; ATR_CMP_REF_PWM input; RA_ON input; LOWER_RATE input; PERIOD input; VENT_CMP_REF_PWM input; time input double [0..]; oldTime constant double =0
